simulink model "check_serial_new_arduino_time"  (R2020b)
settings: Solver=FixedStepDiscrete  StartTime=0.0  StopTime=inf  FixedStep=time_step  RelTol=1e-3
model workspace (MAT data in the model file):
  time_step = 0.01
undefined symbols (not defined in the file or in its folder): DiscIntNeverNeededParam, Serial_Port, Standard_Devices
libraries: sldrtlib x2
settings Model: OrderedModelArguments=off  Creator=Rahul Subramanian  LastModifiedBy=Rahul Subramanian

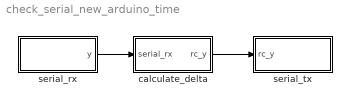
== system check_serial_new_arduino_time ==
  calculate_delta : Subsystem
  serial_rx : Subsystem
  serial_tx : Subsystem
  wires:
  serial_rx/1(y) -> calculate_delta/1(serial_rx)
  calculate_delta/1(rc_y) -> serial_tx/1(rc_y)

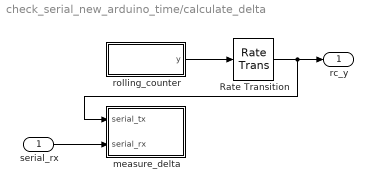
== system check_serial_new_arduino_time/calculate_delta ==
  serial_rx : Inport
  Rate Transition : RateTransition  Integrity=off  Deterministic=off  OutPortSampleTime=time_step
  measure_delta : Subsystem
  rolling_counter : Subsystem
  rc_y : Outport
  wires:
  rolling_counter/1(y) -> Rate Transition/1
  Rate Transition/1 -> rc_y/1, measure_delta/1(serial_tx)
  serial_rx/1 -> measure_delta/2(serial_rx)

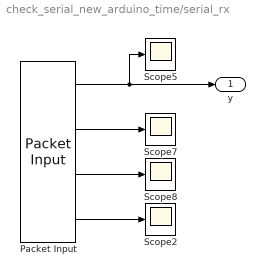
== system check_serial_new_arduino_time/serial_rx ==
  Packet Input : sldrtlib/Packet Input  SampleTime=time_step  MaxMissedTicks=inf  ShowMissedTicks=on  YieldWhenWaiting=off  DrvName=Standard_Devices/Serial_Port  DrvAddress=5  DrvOptions=[115200 8 0 0 0 0 0 0]  PacketSize=1  DataTypes='1*uint8'  ShowReady=on  ShowError=on  PacketID=1  ByteOrder=1  ShowTimestamp=off
      settings: AttributesFormatString=Serial Port [5]
  Scope{2,5,7..8} (4 alike) : Scope
  y : Outport
  wires:
  Packet Input/3 -> Scope8/1
  Packet Input/1 -> y/1, Scope5/1
  Packet Input/4 -> Scope2/1
  Packet Input/2 -> Scope7/1

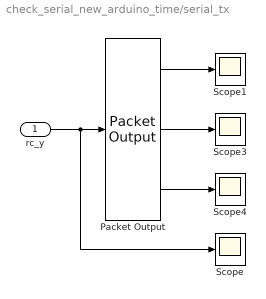
== system check_serial_new_arduino_time/serial_tx ==
  rc_y : Inport
  Packet Output : sldrtlib/Packet Output  SampleTime=time_step  MaxMissedTicks=inf  ShowMissedTicks=on  YieldWhenWaiting=off  DrvName=Standard_Devices/Serial_Port  DrvAddress=5  DrvOptions=[115200 8 0 0 0 0 0 0]  PacketSize=1  DataTypes='1*uint8'  ShowReady=on  ShowError=on  PacketID=1  ByteOrder=1  InitialValue=[]  FinalValue=[]
      settings: AttributesFormatString=Serial Port [5]
  Scope{,1,3..4} (4 alike) : Scope
  wires:
  Packet Output/3 -> Scope4/1
  Packet Output/2 -> Scope3/1
  rc_y/1 -> Scope/1, Packet Output/1
  Packet Output/1 -> Scope1/1

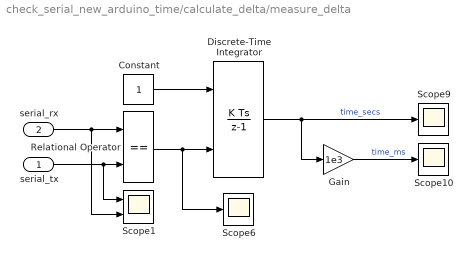
== system check_serial_new_arduino_time/calculate_delta/measure_delta ==
  serial_tx : Inport
  serial_rx : Inport  Port=2
  Constant : Constant
  Discrete-Time Integrator : DiscreteIntegrator  ExternalReset=level  SampleTime=-1  ICPrevOutput=DiscIntNeverNeededParam  ICPrevScaledInput=DiscIntNeverNeededParam
  Gain : Gain  Gain=1e3
  Relational Operator : RelationalOperator  Operator===  OutDataTypeStr=boolean  RndMeth=Simplest
  Scope1 : Scope  NumInputPorts=2
  Scope10 : Scope
  Scope6 : Scope
  Scope9 : Scope
  wires:
  Constant/1 -> Discrete-Time Integrator/1
  Relational Operator/1 -> Scope6/1, Discrete-Time Integrator/2
  serial_tx/1 -> Scope1/1, Relational Operator/2
  serial_rx/1 -> Scope1/2, Relational Operator/1
  Discrete-Time Integrator/1 -> Gain/1, Scope9/1  "time_secs"
  Gain/1 -> Scope10/1  "time_ms"

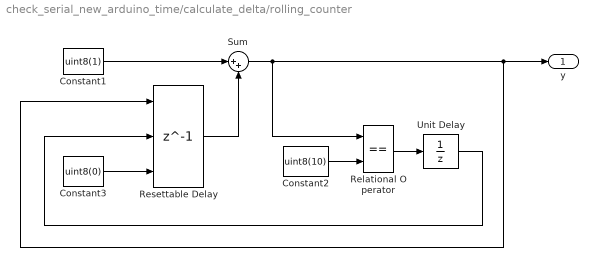
== system check_serial_new_arduino_time/calculate_delta/rolling_counter ==
  Constant1 : Constant  Value=uint8(1)
  Constant2 : Constant  Value=uint8(10)
  Constant3 : Constant  Value=uint8(0)
  Relational O perator : RelationalOperator  Operator===  OutDataTypeStr=boolean  RndMeth=Simplest
  Resettable Delay : Delay  DelayLength=1  InitialConditionSource=Input port  ExternalReset=Rising  SampleTime=0.1
      settings: InputPortMap=u0,r5,p4
  Sum : Sum  Inputs=|++
  Unit Delay : UnitDelay  SampleTime=-1  HasFrameUpgradeWarning=on
  y : Outport
  wires:
  Constant2/1 -> Relational O perator/2
  Constant3/1 -> Resettable Delay/3
  Resettable Delay/1 -> Sum/2
  Sum/1 -> Relational O perator/1, y/1, Resettable Delay/1
  Unit Delay/1 -> Resettable Delay/2
  Constant1/1 -> Sum/1
  Relational O perator/1 -> Unit Delay/1
